simulink model "Battery_Model"  (R2023a)
settings: Solver=ode23tb  StartTime=0.0  StopTime=20000  FixedStep=0.1  MaxStep=0.01  MinStep=0.001  RelTol=1e-3
undefined symbols (not defined in the file or in its folder): Battery_C1, Battery_R1, Battery_Rs, Battery_SOC, Battery_SOC0, Battery_U_OCV
libraries: simulink x1
settings Model: Creator=lucea  LastModifiedBy=gabrielcrisan

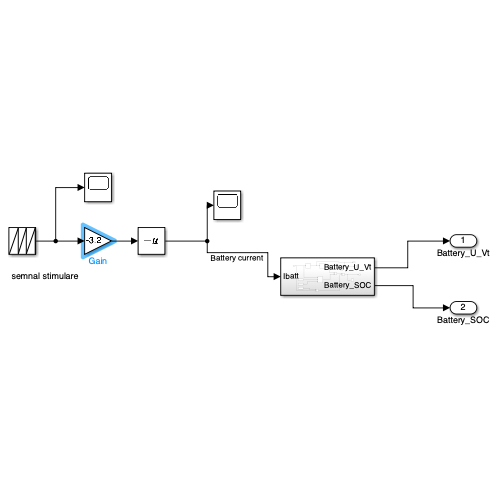
[thumbnail: Simulink's stored preview of the top-level diagram]
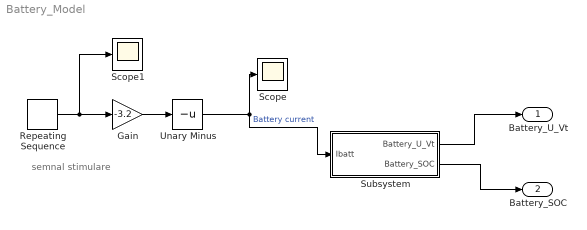
== system Battery_Model ==
  note: semnal stimulare
  Gain : Gain  Gain=-3.2
  Repeating Sequence : simulink/Sources/Repeating Sequence  rep_seq_t=time  rep_seq_y=pulse
  Scope : Scope
  Scope1 : Scope
  Subsystem : Subsystem
  Unary Minus : UnaryMinus
  Battery_U_Vt : Outport
  Battery_SOC : Outport  Port=2
  wires:
  Unary Minus/1 -> Subsystem/1(Ibatt), Scope/1  "Battery current"
  Subsystem/1(Battery_U_Vt) -> Battery_U_Vt/1
  Subsystem/2(Battery_SOC) -> Battery_SOC/1
  Repeating Sequence/1 -> Scope1/1, Gain/1
  Gain/1 -> Unary Minus/1

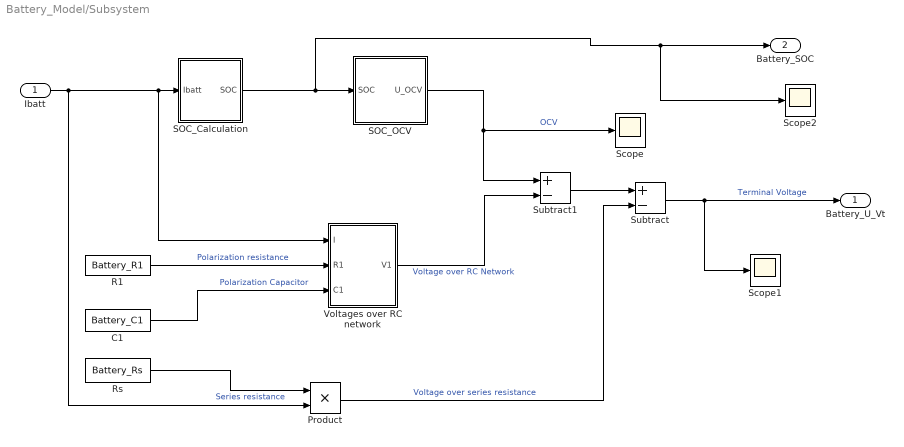
== system Battery_Model/Subsystem ==
  Ibatt : Inport
  C1 : Constant  Value=Battery_C1
  Product : Product
  R1 : Constant  Value=Battery_R1
  Rs : Constant  Value=Battery_Rs
  SOC_Calculation : Subsystem
  SOC_OCV : Subsystem
  Scope : Scope
  Scope1 : Scope
  Scope2 : Scope
  Subtract : Sum  Inputs=+-
  Subtract1 : Sum  Inputs=+-
  Voltages over RC network : Subsystem
  Battery_U_Vt : Outport
  Battery_SOC : Outport  Port=2
  wires:
  Subtract/1 -> Scope1/1, Battery_U_Vt/1  "Terminal Voltage"
  Rs/1 -> Product/1  "Series resistance"
  C1/1 -> Voltages over RC network/3(C1)  "Polarization Capacitor"
  SOC_OCV/1(U_OCV) -> Scope/1, Subtract1/1  "OCV"
  SOC_Calculation/1(SOC) -> Scope2/1, Battery_SOC/1, SOC_OCV/1(SOC)
  Subtract1/1 -> Subtract/1
  Ibatt/1 -> Product/2, Voltages over RC network/1(I), SOC_Calculation/1(Ibatt)
  Voltages over RC network/1(V1) -> Subtract1/2  "Voltage over RC Network"
  R1/1 -> Voltages over RC network/2(R1)  "Polarization resistance"
  Product/1 -> Subtract/2  "Voltage over series resistance"

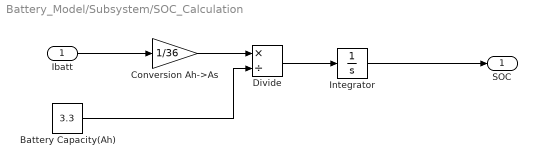
== system Battery_Model/Subsystem/SOC_Calculation ==
  Ibatt : Inport
  Battery Capacity(Ah) : Constant  Value=3.3
  Conversion Ah->As : Gain  Gain=1/36
  Divide : Product  Inputs=*/
  Integrator : Integrator  InitialCondition=Battery_SOC0
  SOC : Outport
  wires:
  Divide/1 -> Integrator/1
  Battery Capacity(Ah)/1 -> Divide/2
  Conversion Ah->As/1 -> Divide/1
  Ibatt/1 -> Conversion Ah->As/1
  Integrator/1 -> SOC/1

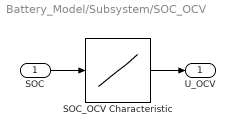
== system Battery_Model/Subsystem/SOC_OCV ==
  SOC : Inport
  SOC_OCV Characteristic : Lookup_n-D  NumberOfTableDimensions=1  BreakpointsForDimension1=Battery_SOC  Table=Battery_U_OCV  InternalRulePriority=Speed  RndMeth=Simplest
  U_OCV : Outport
  wires:
  SOC/1 -> SOC_OCV Characteristic/1
  SOC_OCV Characteristic/1 -> U_OCV/1

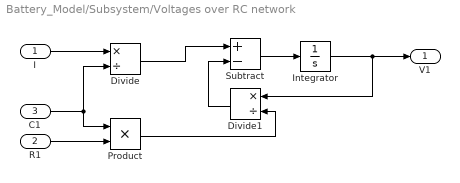
== system Battery_Model/Subsystem/Voltages over RC network ==
  I : Inport
  R1 : Inport  Port=2
  C1 : Inport  Port=3
  Divide : Product  Inputs=*/
  Divide1 : Product  Inputs=*/
  Integrator : Integrator
  Product : Product
  Subtract : Sum  Inputs=+-
  V1 : Outport
  wires:
  R1/1 -> Product/2
  Integrator/1 -> V1/1, Divide1/1
  I/1 -> Divide/1
  Divide/1 -> Subtract/1
  Divide1/1 -> Subtract/2
  C1/1 -> Divide/2, Product/1
  Product/1 -> Divide1/2
  Subtract/1 -> Integrator/1
